simulink model "model"  (R2023a)
settings: Solver=VariableStepAuto  StartTime=0.0  StopTime=10.0  RelTol=1e-3
libraries: BatteryCurrentManagement x2, spsGenericPowerSystemStabilizerLib x1
settings Model: Creator=Pedro  LastModifiedBy=DNS

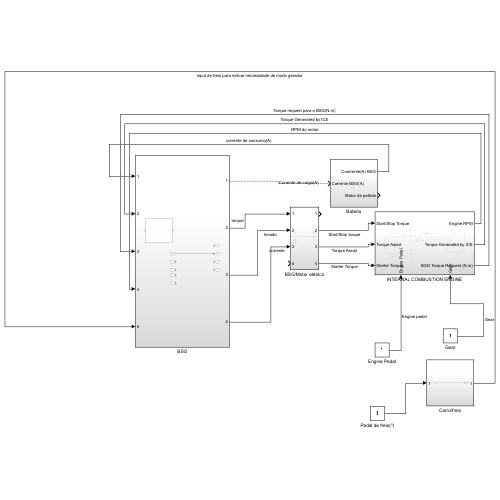
[thumbnail: Simulink's stored preview of the top-level diagram]
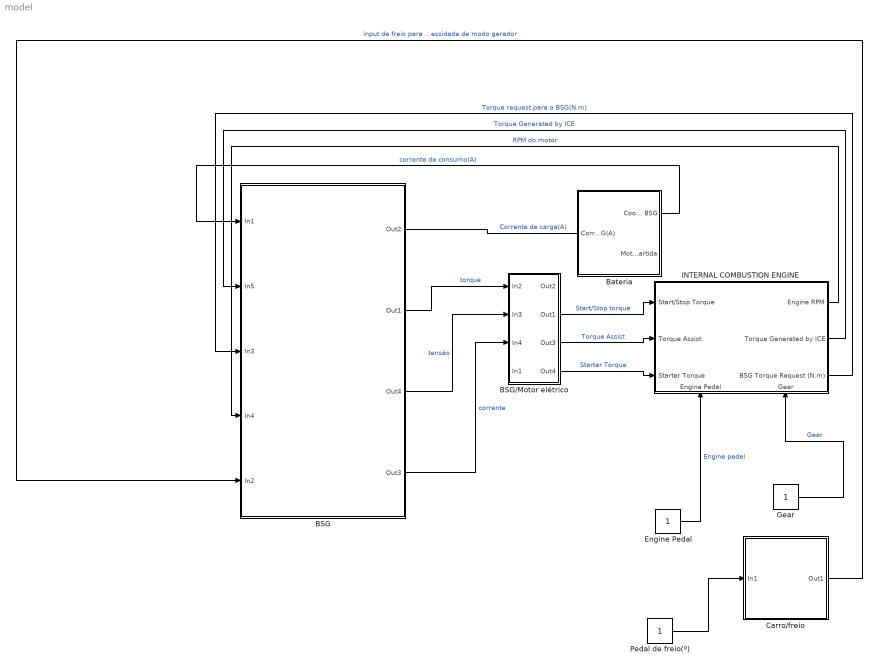
== system model ==
  BSG : Subsystem
  BSG/Motor elétrico : Subsystem
  Bateria : Subsystem
  Carro/freio : Subsystem
  Engine Pedal : Constant
  Gear : Constant
  INTERNAL COMBUSTION ENGINE : Subsystem
      settings: PortSchema="{\"entries\":[{\"content\":{\"sides\":[{\"content\":{\"connectorIds\":[\"In1\",\"In2\",\"In3\"]},\"type\":\"ConnectorPlacement.EquallySpacedRectSide\",\"uuid\":\"ce092393-4b5e-4455-aba9-0cf9705a5882\"},{\"content\":{\"connectorIds\":[\"Out1\",\"Out2\",\"Out3\"],\"side\":\"RIGHT\"},\"type\":\"ConnectorPlacement.EquallySpacedRectSide\",\"uuid\":\"39f1620d-f19f-4d17-9a2c-1204b4040c22\"},{\"content\":{\"side\":\"TOP\"},\"type\":\"ConnectorPlacement.EquallySpacedRectSide\",\"uuid\":\"940edc2a-8e4d-4800-9ba5-7e24d0f8ee78\"},{\"content\":{\"connectorIds\":[\"In4\",\"In5\"],\"side\":\"BOTTOM\"},\"type\":\"ConnectorPlacement.EquallySpacedRectSide\",\"uuid\":\"a8c92029-a525-4a44-9138-e7028dc0182e\"}]},\"type\":\"ConnectorPlacement.EquallySpacedConnector\",\"uuid\":\"b09c41f2-a1e2-4cd1-915a-dc8e84f252cd\"}],\"packageUris\":[\"http://schema.mathworks.com/mf0/Connector/R2020b\"],\"version\":\"1.0\"}"
  Pedal de freio(º) : Constant
  wires:
  BSG/1(Out2) -> ?  "Corrente de carga(A)"
  Bateria/1(Coorrente(A) BSG) -> BSG/1(In1)  "corrente de consumo(A)"
  Engine Pedal/1 -> INTERNAL COMBUSTION ENGINE/4(Engine Pedal)  "Engine pedal"
  Pedal de freio(º)/1 -> Carro/freio/1(In1)
  Carro/freio/1(Out1) -> BSG/5(In2)  "input de freio para indicar necessidade de modo gerador"
  Gear/1 -> INTERNAL COMBUSTION ENGINE/5(Gear)  "Gear"
  INTERNAL COMBUSTION ENGINE/3(BSG Torque Request (N.m)) -> BSG/3(In3)  "Torque request para o BSG(N.m)"
  INTERNAL COMBUSTION ENGINE/1(Engine RPM) -> BSG/4(In4)  "RPM do motor"
  INTERNAL COMBUSTION ENGINE/2(Torque Generated by ICE) -> BSG/2(In5)  "Torque Generated by ICE"
  BSG/Motor elétrico/2(Out1) -> INTERNAL COMBUSTION ENGINE/1(Start/Stop Torque)  "Start/Stop torque"
  BSG/2(Out1) -> BSG/Motor elétrico/1(In2)  "torque"
  BSG/3(Out4) -> BSG/Motor elétrico/2(In3)  "tensão"
  BSG/4(Out3) -> BSG/Motor elétrico/3(In4)  "corrente"
  BSG/Motor elétrico/3(Out3) -> INTERNAL COMBUSTION ENGINE/2(Torque Assist)  "Torque Assist"
  BSG/Motor elétrico/4(Out4) -> INTERNAL COMBUSTION ENGINE/3(Starter Torque)  "Starter Torque"

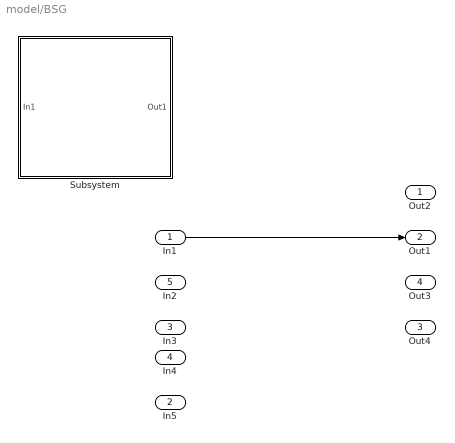
== system model/BSG ==
  In1 : Inport
  In5 : Inport  Port=2
  In3 : Inport  Port=3
  In4 : Inport  Port=4
  In2 : Inport  Port=5
  Subsystem : Subsystem
  Out2 : Outport
  Out1 : Outport  Port=2
  Out4 : Outport  Port=3
  Out3 : Outport  Port=4
  wires:
  In1/1 -> Out1/1

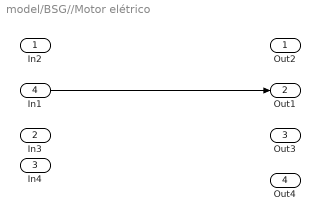
== system model/BSG//Motor elétrico ==
  In2 : Inport
  In3 : Inport  Port=2
  In4 : Inport  Port=3
  In1 : Inport  Port=4
  Out2 : Outport
  Out1 : Outport  Port=2
  Out3 : Outport  Port=3
  Out4 : Outport  Port=4
  wires:
  In1/1 -> Out1/1

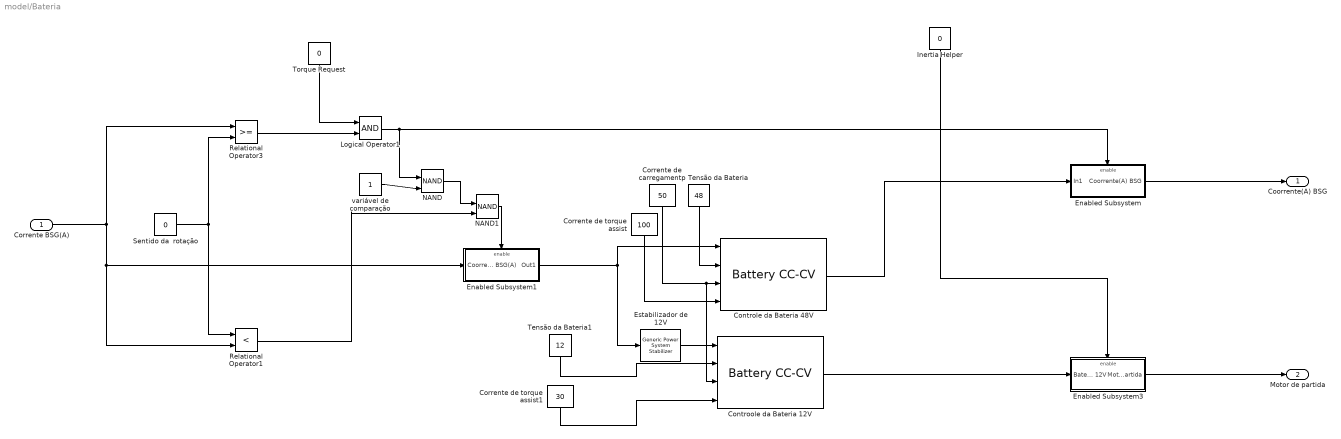
== system model/Bateria ==
  Corrente BSG(A) : Inport
  " Inertia Helper" : Constant  Value=0
  Controle da Bateria 48V : BatteryCurrentManagement/Battery CC-CV  MaxCellVoltage=48  Kp=100  Ki=10  Kaw=1  Kt=1  Ts=1
      settings: LibrarySourceBlock=batt_sl_lib/Current Management/Battery CC-CV
  Controole da Bateria 12V : BatteryCurrentManagement/Battery CC-CV  MaxCellVoltage=12  Kp=100  Ki=10  Kaw=1  Kt=1  Ts=1
      settings: LibrarySourceBlock=batt_sl_lib/Current Management/Battery CC-CV
  Corrente de carregamentp : Constant  Value=50
  Corrente de torque assist : Constant  Value=100
  Corrente de torque assist1 : Constant  Value=30
  Enabled Subsystem : Subsystem  TreatAsAtomicUnit=on
  Enabled Subsystem1 : Subsystem  TreatAsAtomicUnit=on
  Enabled Subsystem3 : Subsystem  TreatAsAtomicUnit=on
  "Estabilizador de 12V " : spsGenericPowerSystemStabilizerLib/Generic Power System Stabilizer  Tsensor=30e-3  K=20  Twashout=2  Tleadlag1=[50e-3 20e-3]  Tleadlag2=[3 5.4]  VSlimits=[12 12.10]  Vinit=0  Plot_On=off  MagdB_On=on  FreqRange=logspace(-2,2,500)
      settings: LibrarySourceBlock=|
      | sps_lib/Electrical Machines/Synchronous Machine Control/Generic
      | Power System Stabilizer
  Logical Operator1 : Logic  AllPortsSameDT=off  OutDataTypeStr=boolean
  NAND : Logic  Operator=NAND  IconShape=distinctive  AllPortsSameDT=off  OutDataTypeStr=boolean
  NAND1 : Logic  Operator=NAND  IconShape=distinctive  AllPortsSameDT=off  OutDataTypeStr=boolean
  Relational Operator1 : RelationalOperator  Operator=<  OutDataTypeStr=boolean  RndMeth=Simplest  InputSameDT=off
  Relational Operator3 : RelationalOperator  OutDataTypeStr=boolean  RndMeth=Simplest  InputSameDT=off
  Sentido da  rotação : Constant  Value=0
  Tensão da Bateria : Constant  Value=48
  Tensão da Bateria1 : Constant  Value=12
  Torque Request : Constant  Value=0
  variável de comparação : Constant
  Coorrente(A) BSG : Outport
  Motor de partida : Outport  Port=2
  wires:
  Corrente BSG(A)/1 -> Enabled Subsystem1/1(Coorrente BSG(A)), Relational Operator1/2, Relational Operator3/1
  Sentido da  rotação/1 -> Relational Operator3/2, Relational Operator1/1
  Relational Operator3/1 -> Logical Operator1/2
  Torque Request/1 -> Logical Operator1/1
  Logical Operator1/1 -> NAND/1, Enabled Subsystem/Enable
  variável de comparação/1 -> NAND/2
  Controle da Bateria 48V/1 -> Enabled Subsystem/1(In1)
  Enabled Subsystem/1(Coorrente(A) BSG) -> Coorrente(A) BSG/1
  " Inertia Helper"/1 -> Enabled Subsystem3/Enable
  Controole da Bateria 12V/1 -> Enabled Subsystem3/1(Bateria 12V)
  Enabled Subsystem1/1(Out1) -> Controle da Bateria 48V/1, "Estabilizador de 12V "/1
  NAND/1 -> NAND1/1
  NAND1/1 -> Enabled Subsystem1/Enable
  Relational Operator1/1 -> NAND1/2
  "Estabilizador de 12V "/1 -> Controole da Bateria 12V/1
  Tensão da Bateria1/1 -> Controole da Bateria 12V/2
  Tensão da Bateria/1 -> Controle da Bateria 48V/2
  Corrente de carregamentp/1 -> Controole da Bateria 12V/3, Controle da Bateria 48V/3
  Corrente de torque assist/1 -> Controle da Bateria 48V/4
  Corrente de torque assist1/1 -> Controole da Bateria 12V/4
  Enabled Subsystem3/1(Motor de partida) -> Motor de partida/1

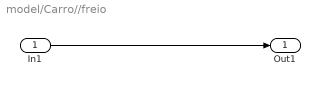
== system model/Carro//freio ==
  In1 : Inport
  Out1 : Outport
  wires:
  In1/1 -> Out1/1

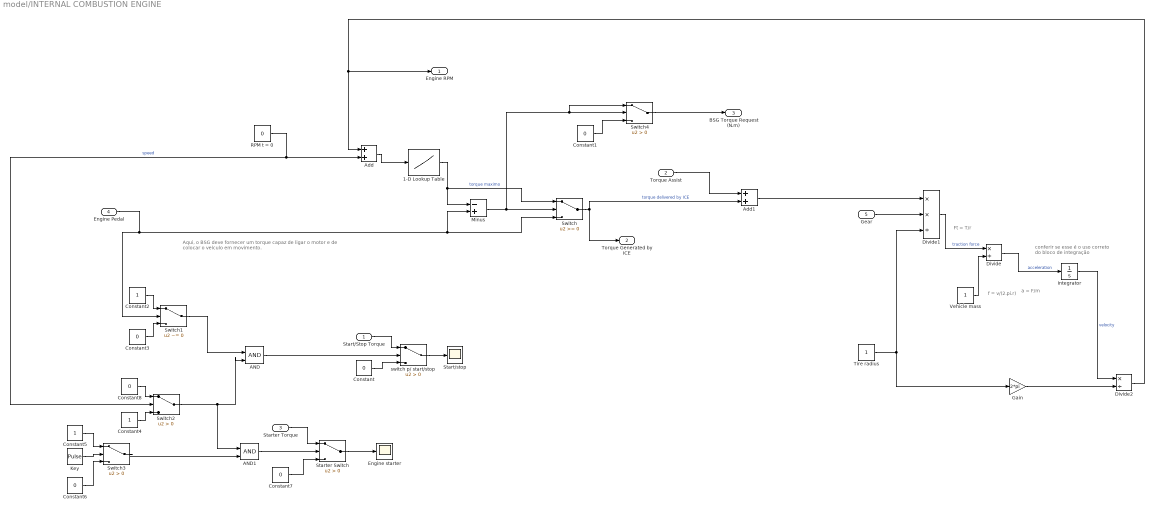
== system model/INTERNAL COMBUSTION ENGINE ==
  note: a = F/m
  note: f = v/(2.pi.r)
  note: Ft = T/r
  note: conferir se esse é o uso
      | correto do bloco de integração
  note: Aqui, o BSG deve fornecer um torque capaz de ligar o motor e
      | de colocar o veículo em movimento.
  Start/Stop Torque : Inport
  Torque Assist : Inport  Port=2
  Starter Torque : Inport  Port=3
  Engine Pedal : Inport  Port=4
  Gear : Inport  Port=5
  1-D Lookup Table : Lookup_n-D  NumberOfTableDimensions=1  BreakpointsForDimension1=[-5:5]  Table=tanh([-5:5])  InternalRulePriority=Speed  RndMeth=Simplest
  AND : Logic  IconShape=distinctive  AllPortsSameDT=off  OutDataTypeStr=boolean
  AND1 : Logic  IconShape=distinctive  AllPortsSameDT=off  OutDataTypeStr=boolean
  Add : Sum
  Add1 : Sum
  Constant{,1,3,6..8} (6 alike) : Constant  Value=0
  Constant2 : Constant
  Constant4 : Constant
  Constant5 : Constant
  Divide : Product  Inputs=*/
  Divide1 : Product  Inputs=**/
  Divide2 : Product  Inputs=*/
  Engine starter : Scope
  Gain : Gain  Gain=2*pi
  Integrator : Integrator
  Key : DiscretePulseGenerator  PulseType=Time based  Period=1  PulseWidth=5
  Minus : Sum  Inputs=-+
  RPM t = 0 : Constant  Value=0
  Start/stop : Scope
  Starter Switch : Switch  Criteria=u2 > Threshold  SaturateOnIntegerOverflow=off  InputSameDT=off
  Switch : Switch  SaturateOnIntegerOverflow=off  InputSameDT=off
  Switch1 : Switch  Criteria=u2 ~= 0  SaturateOnIntegerOverflow=off  InputSameDT=off
  Switch2 : Switch  Criteria=u2 > Threshold  SaturateOnIntegerOverflow=off  InputSameDT=off
  Switch3 : Switch  Criteria=u2 > Threshold  SaturateOnIntegerOverflow=off  InputSameDT=off
  Switch4 : Switch  Criteria=u2 > Threshold  SaturateOnIntegerOverflow=off  InputSameDT=off
  Tire radius : Constant
  Vehicle mass : Constant
  switch p/ start/stop : Switch  Criteria=u2 > Threshold  SaturateOnIntegerOverflow=off  InputSameDT=off
  Engine RPM : Outport
  Torque Generated by ICE : Outport  Port=2
  BSG Torque Request (N.m) : Outport  Port=3
  wires:
  AND/1 -> switch p/ start/stop/2
  RPM t = 0/1 -> Add/2, Switch2/2  "speed"
  1-D Lookup Table/1 -> Switch/1, Minus/1  "torque maximo"
  Engine Pedal/1 -> Switch1/2, Switch/3, Minus/2
  Constant5/1 -> Switch3/1
  Constant2/1 -> Switch1/1
  Switch2/1 -> AND1/1, AND/2
  Constant3/1 -> Switch1/3
  Switch/1 -> Add1/2, Torque Generated by ICE/1  "torque delivered by ICE"
  Vehicle mass/1 -> Divide/2
  Minus/1 -> Switch4/1, Switch4/2, Switch/2
  Add/1 -> 1-D Lookup Table/1
  Start/Stop Torque/1 -> switch p/ start/stop/1
  Constant/1 -> switch p/ start/stop/3
  Switch3/1 -> AND1/2
  Gain/1 -> Divide2/2
  Divide/1 -> Integrator/1  "acceleration"
  Tire radius/1 -> Divide1/3, Gain/1
  Divide1/1 -> Divide/1  "traction force"
  switch p/ start/stop/1 -> Start/stop/1
  Key/1 -> Switch3/2
  Divide2/1 -> Add/1, Engine RPM/1
  Integrator/1 -> Divide2/1  "velocity"
  AND1/1 -> Starter Switch/2
  Constant6/1 -> Switch3/3
  Switch1/1 -> AND/1
  Constant4/1 -> Switch2/3
  Constant1/1 -> Switch4/3
  Switch4/1 -> BSG Torque Request (N.m)/1
  Torque Assist/1 -> Add1/1
  Add1/1 -> Divide1/1
  Gear/1 -> Divide1/2
  Starter Torque/1 -> Starter Switch/1
  Constant7/1 -> Starter Switch/3
  Constant8/1 -> Switch2/1
  Starter Switch/1 -> Engine starter/1

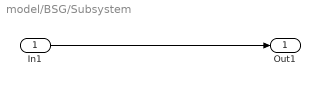
== system model/BSG/Subsystem ==
  In1 : Inport
  Out1 : Outport
  wires:
  In1/1 -> Out1/1

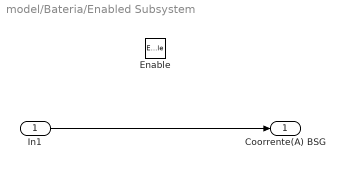
== system model/Bateria/Enabled Subsystem ==
  In1 : Inport
  Enable : EnablePort
  Coorrente(A) BSG : Outport
  wires:
  In1/1 -> Coorrente(A) BSG/1

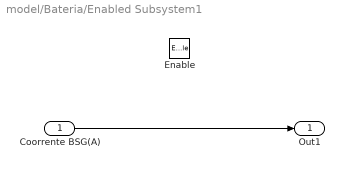
== system model/Bateria/Enabled Subsystem1 ==
  Coorrente BSG(A) : Inport
  Enable : EnablePort
  Out1 : Outport
  wires:
  Coorrente BSG(A)/1 -> Out1/1

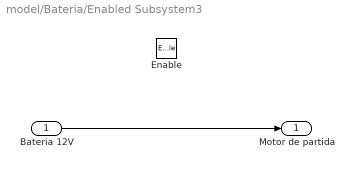
== system model/Bateria/Enabled Subsystem3 ==
  Bateria 12V : Inport
  Enable : EnablePort
  Motor de partida : Outport
  wires:
  Bateria 12V/1 -> Motor de partida/1
